simulink model "MSFartoystyring"  (Simulink 8.6)
settings: Solver=ode45  StartTime=tstart  StopTime=tstop  RelTol=1e-3
values from neighbouring files (symbols this model uses):
  c = 0    [run.m]
  Kd = 0    [run.m]
  Ki = 0    [run.m]
  Ki_speed = 0    [run.m]
  Kp = 10    [run.m]
  Kp_speed = 0    [run.m]
  psi0 = 0    [run.m]
  r0 = 0    [run.m]
  tsamp = 10    [run.m]
  v0 = [6.63 0]'    [run.m]
undefined symbols (not defined in the file or in its folder): msfartoystyring, WP
undefined symbols (not defined in the file): p0
settings Model: Creator=christh  LastModifiedBy=Arne Selle  ExtModeAutoUpdateStatusClock=off
settings OptimizationCC: InitFltsAndDblsToZero=on
settings DebuggingCC: FcnCallInpInsideContextMsg=UseLocalSettings

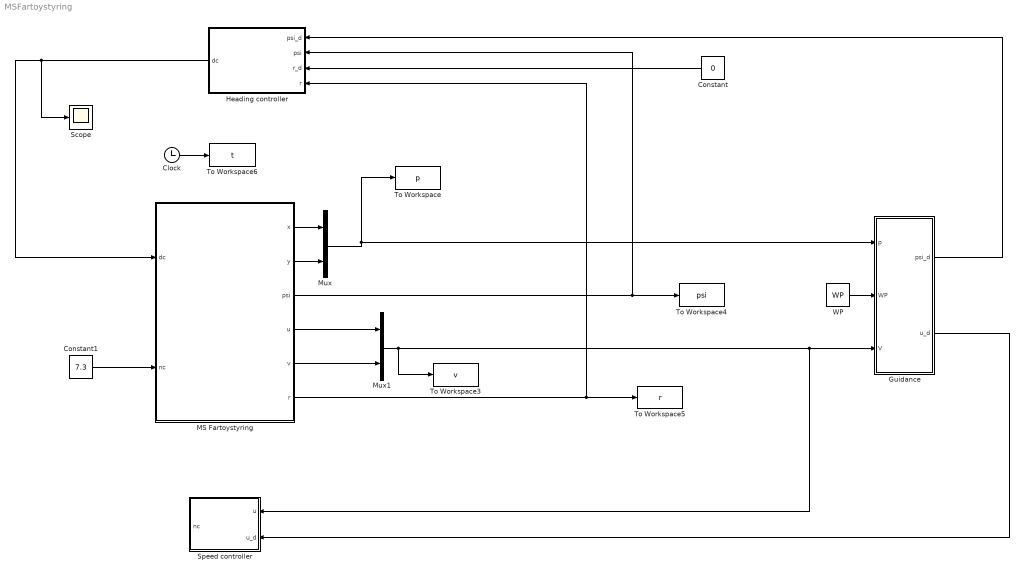
== system MSFartoystyring ==
  Clock : Clock
  Constant : Constant  Value=0
  Constant1 : Constant  Value=7.3
  Guidance : Subsystem
  Heading controller : Subsystem
  MS Fartoystyring : Subsystem  mask(MS Fartoystyring for Assignment 3 G&C){x0=p0(1), y0=p0(2), u0=v0(1), v0=v0(2), psi0=psi0, r0=r0, c=c}
      mask prompts: x0 "x(t0) (m)"; y0 "y(t0) (m)"; u0 "u(t0) (m/s)"; v0 "v(t0) (m/s)"; psi0 "psi(t0) (rad)"; r0 "r(t0) (rad/s)"; c "current (0 or 1)"
      mask help:
      | Block corresponding to Figure 1 in the assignment text. Gives the response of the ship.
      |
      | The design speed of MS Fartoystyring is u=8.23 m/s.
      |
      | Input:
      | dc: commanded rudder (rad), dmax=25*pi/180
      | nc: commanded shaft speed (rad/s), nmax=85*2*pi/60
      |
      | Output:
      | x: north pos (m)
      | y: east pos (m)
      | u: surge (m/s)
      | v: sway (m/s)
      | psi: heading (rad)
      | r: yaw (rad/s)
      mask Help: Comments, bugs and help requests can be directed to the TA. Email on course website.
  Mux : Mux  Inputs=2
  Mux1 : Mux  Inputs=2
  Scope : Scope
  Speed controller : Subsystem
  To Workspace : ToWorkspace  VariableName=p  SampleTime=tsamp
  To Workspace3 : ToWorkspace  VariableName=v  SampleTime=tsamp
  To Workspace4 : ToWorkspace  VariableName=psi  SampleTime=tsamp
  To Workspace5 : ToWorkspace  VariableName=r  SampleTime=tsamp
  To Workspace6 : ToWorkspace  VariableName=t  SampleTime=tsamp
  WP : Constant  Value=WP
  wires:
  Clock/1 -> To Workspace6/1
  MS Fartoystyring/1(x) -> Mux/1
  MS Fartoystyring/2(y) -> Mux/2
  MS Fartoystyring/4(u) -> Mux1/1
  MS Fartoystyring/5(v) -> Mux1/2
  Mux/1 -> Guidance/1(p), To Workspace/1
  MS Fartoystyring/3(psi) -> Heading controller/2(psi), To Workspace4/1
  MS Fartoystyring/6(r) -> Heading controller/4(r), To Workspace5/1
  Heading controller/1(dc) -> Scope/1, MS Fartoystyring/1(dc)
  Mux1/1 -> To Workspace3/1, Speed controller/1(u), Guidance/3(V)
  Guidance/1(psi_d) -> Heading controller/1(psi_d)
  Guidance/2(u_d) -> Speed controller/2(u_d)
  Constant/1 -> Heading controller/3(r_d)
  WP/1 -> Guidance/2(WP)
  Constant1/1 -> MS Fartoystyring/2(nc)

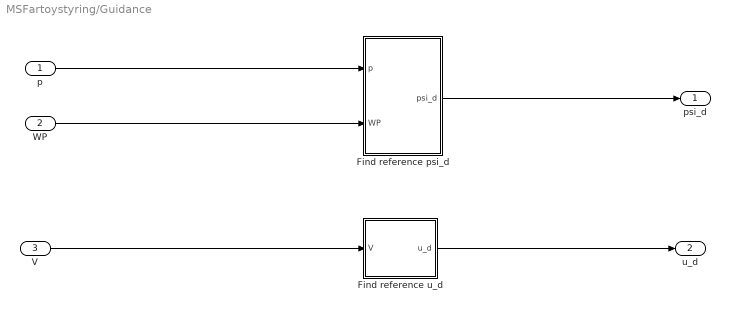
== system MSFartoystyring/Guidance ==
  p : Inport
  WP : Inport  Port=2
  V : Inport  Port=3
  Find reference psi_d : MATLAB Function  TreatAsAtomicUnit=on
  Find reference u_d : MATLAB Function  TreatAsAtomicUnit=on
  psi_d : Outport
  u_d : Outport  Port=2
  wires:
  V/1 -> Find reference u_d/1(V)
  Find reference u_d/1(u_d) -> u_d/1
  p/1 -> Find reference psi_d/1(p)
  WP/1 -> Find reference psi_d/2(WP)
  Find reference psi_d/1(psi_d) -> psi_d/1

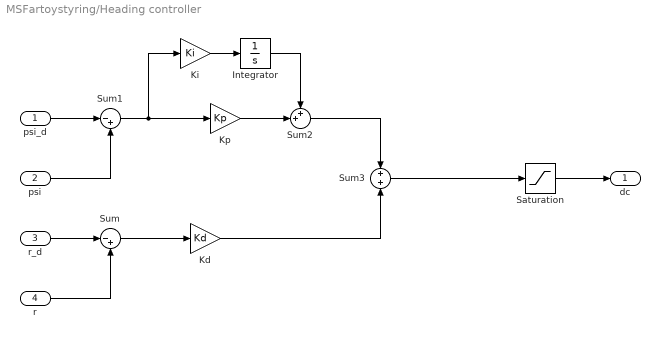
== system MSFartoystyring/Heading controller ==
  psi_d : Inport
  psi : Inport  Port=2
  r_d : Inport  Port=3
  r : Inport  Port=4
  Integrator : Integrator
  Kd : Gain  Gain=Kd
  Ki : Gain  Gain=Ki
  Kp : Gain  Gain=Kp
  Saturation : Saturate  UpperLimit=deg2rad(25)  LowerLimit=-deg2rad(25)
  Sum : Sum  Inputs=|-+
  Sum1 : Sum  Inputs=|-+
  Sum2 : Sum  Inputs=++|
  Sum3 : Sum  Inputs=+|+
  dc : Outport
  wires:
  Sum/1 -> Kd/1
  r/1 -> Sum/2
  r_d/1 -> Sum/1
  psi_d/1 -> Sum1/1
  psi/1 -> Sum1/2
  Sum1/1 -> Ki/1, Kp/1
  Kp/1 -> Sum2/2
  Ki/1 -> Integrator/1
  Kd/1 -> Sum3/2
  Sum3/1 -> Saturation/1
  Sum2/1 -> Sum3/1
  Saturation/1 -> dc/1
  Integrator/1 -> Sum2/1

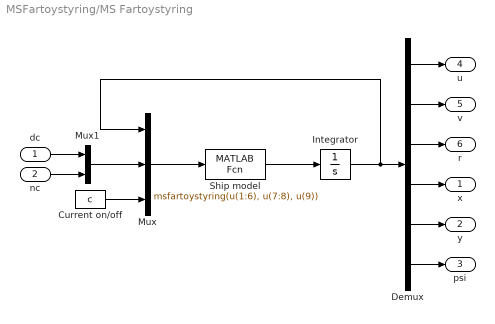
== system MSFartoystyring/MS Fartoystyring ==
  dc : Inport
  nc : Inport  Port=2
  Current on/off : Constant  Value=c
  Demux : Demux  Outputs=6
  Integrator : Integrator  InitialCondition=[u0 v0 r0 x0 y0 psi0]'
  Mux : Mux  Inputs=3
  Mux1 : Mux  Inputs=2
  Ship model : MATLABFcn  MATLABFcn=msfartoystyring(u(1:6), u(7:8), u(9))  OutputDimensions=6
  x : Outport
  y : Outport  Port=2
  psi : Outport  Port=3
  u : Outport  Port=4
  v : Outport  Port=5
  r : Outport  Port=6
  wires:
  Integrator/1 -> Mux/1, Demux/1
  Mux1/1 -> Mux/2
  dc/1 -> Mux1/1
  nc/1 -> Mux1/2
  Demux/1 -> u/1
  Demux/2 -> v/1
  Demux/3 -> r/1
  Demux/4 -> x/1
  Demux/5 -> y/1
  Demux/6 -> psi/1
  Current on/off/1 -> Mux/3
  Ship model/1 -> Integrator/1
  Mux/1 -> Ship model/1

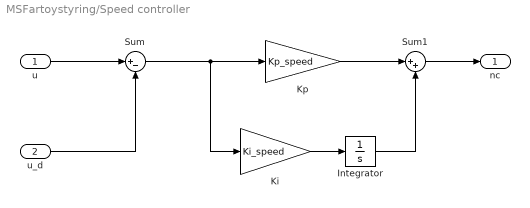
== system MSFartoystyring/Speed controller ==
  u : Inport
  u_d : Inport  Port=2
  Integrator : Integrator
  Ki : Gain  Gain=Ki_speed
  Kp : Gain  Gain=Kp_speed
  Sum : Sum  Inputs=|+-
  Sum1 : Sum  Inputs=|++
  nc : Outport
  wires:
  u_d/1 -> Sum/2
  u/1 -> Sum/1
  Sum/1 -> Ki/1, Kp/1
  Ki/1 -> Integrator/1
  Integrator/1 -> Sum1/2
  Kp/1 -> Sum1/1
  Sum1/1 -> nc/1

== matlab function Guidance/Find reference u_d ==
  data: V input double; u_d output double
function u_d = fcn(V)
%u_d finding reference speed

u_d = sqrt(V(1)^2 + V(2)^2);
end

== matlab function Guidance/Find reference psi_d ==
  data: p input double; psi_d output double; WP input double
function psi_d = fcn(p, WP)
%Finding the reference angle psi_d

persistent index;

if isempty(index)
     index = 2;
end

x = p(1);
y = p(2);

ylos = 0;
xlos = 0;

xk = WP(1, index-1);
yk = WP(2, index-1);

xk_1 = WP(1, index);
yk_1 = WP(2, index);

if (xk_1 - x < 0) && (yk_1 - y > 0) && (length(WP) > index)
    index = index + 1;
end

deltaX = xk_1 - xk;
deltaY = yk_1 - yk;

R2 = (xk_1 - x)^2 + (yk_1 - y)^2;

% case 1
if abs(deltaX) > 0
    d = deltaY / deltaX;
    e = xk;
    f = yk;
    
    g = f - d*e;
    
    a = 1 + d^2;
    b = 2 * (d*g - d*y - x);
    c = x^2 + y^2 + g^2 - 2*g*y - R2;
   
    if deltaX > 0
        xlos = (-b + sqrt(b^2 - 4*a*c)) / (2*a);
        ylos = d * (xlos - xk) + yk;
    else
        xlos = (-b - sqrt(b^2 - 4*a*c)) / (2*a);
        ylos = d * (xlos - xk) + yk;
    end
    
else
    xlos = xk;
    
    if yk > 0
        ylos = y + sqrt(R2 - (xlos - x)^2);
    else
        ylos = y - sqrt(R2 - (xlos - x)^2);
    end
end

% a = atan2(WP(2,index)-p(2), WP(1,index)-p(1)) * 180 / pi

psi_d = atan2(ylos - y, xlos - x);

end
